simulink model "pacemaker_basic_model"  (R2020b)
settings: Solver=FixedStepAuto  StartTime=0.0  StopTime=10.0  FixedStep=1E-3  RelTol=1e-3  EnableMultiTasking=on
undefined symbols (not defined in the file): D0, D1, D10, D11, D12, D13, D2, D3, D4, D5, D6, D7, D8, D9, PTA0, PTA1, PTA2, PTB23, PTB9, PTC16, PTC17, PTC2, PTC3, PTC4, PTD0, PTD1, PTD2, PTD3
libraries: frdmk64flib x16
settings Model: ExtModeTrigDuration=5  Creator=Owner  LastModifiedBy=Anna
settings OptimizationCC: EnhancedBackFolding=on  PassReuseOutputArgsAs=Individual arguments  ZeroExternalMemoryAtStartup=off  ZeroInternalMemoryAtStartup=off  MaxStackSize=64  OptimizeBlockOrder=speed  DifferentSizesBufferReuse=on  OptimizationCustomize=off  EfficientTunableParamExpr=on
settings DebuggingCC: ParameterTunabilityLossMsg=error
settings HardwareCC: ProdBitPerPointer=32  ProdBitPerSizeT=32  ProdBitPerPtrDiffT=32  ProdLargestAtomicInteger=Long  ProdLargestAtomicFloat=Double  ProdWordSize=32  ProdHWDeviceType=ARM Compatible->ARM Cortex
settings SFSimCC: MATLABDynamicMemAlloc=off
settings RTWCC: Description=Embedded Coder  SystemTargetFile=ert.tlc  HardwareBoard=NXP FRDM-K64F  TLCOptions="-aInlineSetEventsForThisBaseRateFcn=TLC_FALSE -aSuppressMultiTaskScheduler=TLC_FALSE  -aRateBasedStepFcn=0"  TemplateMakefile=ert_default_tmf  Toolchain=GNU Tools for ARM Embedded Processors
settings CodeAppCC: ForceParamTrailComments=on  IgnoreCustomStorageClasses=off  OperatorAnnotations=on  SimulinkDataObjDesc=on  SFDataObjDesc=on  InsertBlockDesc=on
settings ERTTargetCC: ExtModeTransport=4  ExtModeMexFile=sendToCommService

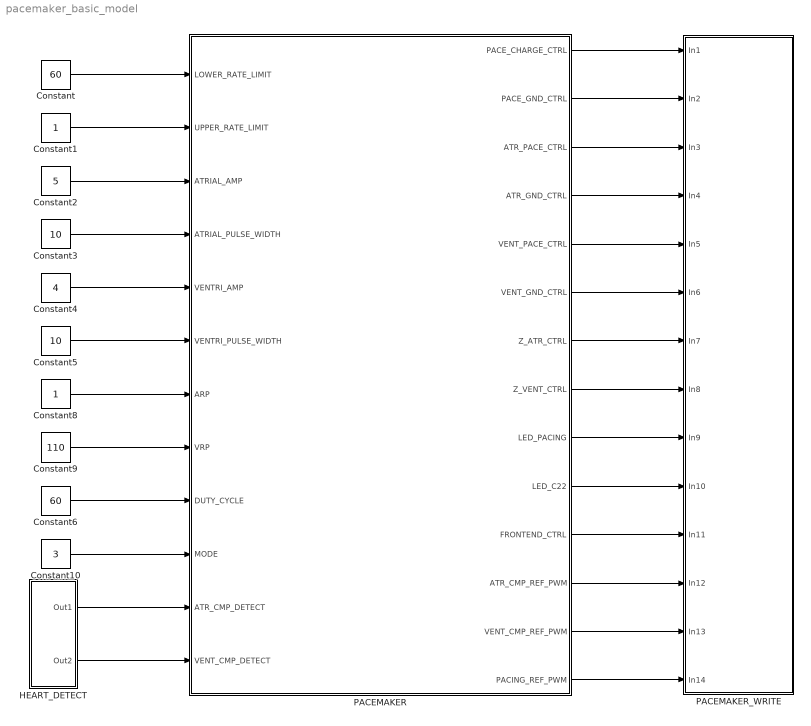
== system pacemaker_basic_model ==
  Constant : Constant  Value=60
  Constant1 : Constant
  Constant10 : Constant  Value=3
  Constant2 : Constant  Value=5
  Constant3 : Constant  Value=10
  Constant4 : Constant  Value=4
  Constant5 : Constant  Value=10
  Constant6 : Constant  Value=60
  Constant8 : Constant
  Constant9 : Constant  Value=110
  HEART_DETECT : Subsystem
  PACEMAKER : Stateflow chart  TreatAsAtomicUnit=on
  PACEMAKER_WRITE : Subsystem
  wires:
  Constant/1 -> PACEMAKER/1(LOWER_RATE_LIMIT)
  Constant1/1 -> PACEMAKER/2(UPPER_RATE_LIMIT)
  Constant2/1 -> PACEMAKER/3(ATRIAL_AMP)
  Constant3/1 -> PACEMAKER/4(ATRIAL_PULSE_WIDTH)
  Constant4/1 -> PACEMAKER/5(VENTRI_AMP)
  Constant5/1 -> PACEMAKER/6(VENTRI_PULSE_WIDTH)
  Constant8/1 -> PACEMAKER/7(ARP)
  Constant9/1 -> PACEMAKER/8(VRP)
  Constant10/1 -> PACEMAKER/10(MODE)
  Constant6/1 -> PACEMAKER/9(DUTY_CYCLE)
  PACEMAKER/1(PACE_CHARGE_CTRL) -> PACEMAKER_WRITE/1(In1)
  PACEMAKER/2(PACE_GND_CTRL) -> PACEMAKER_WRITE/2(In2)
  PACEMAKER/3(ATR_PACE_CTRL) -> PACEMAKER_WRITE/3(In3)
  PACEMAKER/4(ATR_GND_CTRL) -> PACEMAKER_WRITE/4(In4)
  PACEMAKER/5(VENT_PACE_CTRL) -> PACEMAKER_WRITE/5(In5)
  PACEMAKER/6(VENT_GND_CTRL) -> PACEMAKER_WRITE/6(In6)
  PACEMAKER/7(Z_ATR_CTRL) -> PACEMAKER_WRITE/7(In7)
  PACEMAKER/8(Z_VENT_CTRL) -> PACEMAKER_WRITE/8(In8)
  PACEMAKER/9(LED_PACING) -> PACEMAKER_WRITE/9(In9)
  PACEMAKER/10(LED_C22) -> PACEMAKER_WRITE/10(In10)
  PACEMAKER/11(FRONTEND_CTRL) -> PACEMAKER_WRITE/11(In11)
  PACEMAKER/12(ATR_CMP_REF_PWM) -> PACEMAKER_WRITE/12(In12)
  PACEMAKER/13(VENT_CMP_REF_PWM) -> PACEMAKER_WRITE/13(In13)
  PACEMAKER/14(PACING_REF_PWM) -> PACEMAKER_WRITE/14(In14)
  HEART_DETECT/1(Out1) -> PACEMAKER/11(ATR_CMP_DETECT)
  HEART_DETECT/2(Out2) -> PACEMAKER/12(VENT_CMP_DETECT)

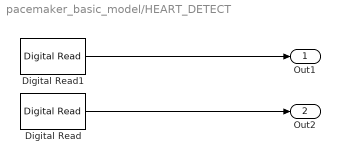
== system pacemaker_basic_model/HEART_DETECT ==
  Digital Read : frdmk64flib/Digital Read  Whichpin=PTC17 (D1)  SampleTime=-1
  Digital Read1 : frdmk64flib/Digital Read  Whichpin=PTC16 (D0)  SampleTime=-1
  Out1 : Outport
  Out2 : Outport  Port=2
  wires:
  Digital Read/1 -> Out2/1
  Digital Read1/1 -> Out1/1

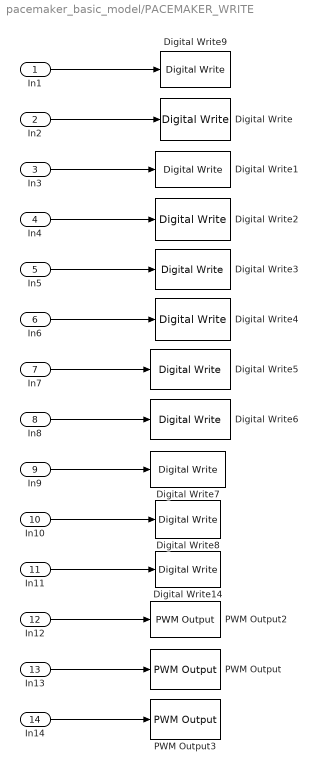
== system pacemaker_basic_model/PACEMAKER_WRITE ==
  In1 : Inport
  In2 : Inport  Port=2
  In3 : Inport  Port=3
  In4 : Inport  Port=4
  In5 : Inport  Port=5
  In6 : Inport  Port=6
  In7 : Inport  Port=7
  In8 : Inport  Port=8
  In9 : Inport  Port=9
  In10 : Inport  Port=10
  In11 : Inport  Port=11
  In12 : Inport  Port=12
  In13 : Inport  Port=13
  In14 : Inport  Port=14
  Digital Write : frdmk64flib/Digital Write  Whichpin=PTD0 (D10)
  Digital Write1 : frdmk64flib/Digital Write  Whichpin=PTA0 (D8)
  Digital Write14 : frdmk64flib/Digital Write  Whichpin=PTD1 (D13)
  Digital Write2 : frdmk64flib/Digital Write  Whichpin=PTD2 (D11)
  Digital Write3 : frdmk64flib/Digital Write  Whichpin=PTC4 (D9)
  Digital Write4 : frdmk64flib/Digital Write  Whichpin=PTD3 (D12)
  Digital Write5 : frdmk64flib/Digital Write  Whichpin=PTB23 (D4)
  Digital Write6 : frdmk64flib/Digital Write  Whichpin=PTC3 (D7)
  Digital Write7 : frdmk64flib/Digital Write  Whichpin=RED_LED
  Digital Write8 : frdmk64flib/Digital Write  Whichpin=BLUE_LED
  Digital Write9 : frdmk64flib/Digital Write  Whichpin=PTB9 (D2)
  PWM Output : frdmk64flib/PWM Output  Whichpin=PTA1 (D3)  InitialFrequency=2000  InitialDutyCycle=100
  PWM Output2 : frdmk64flib/PWM Output  Whichpin=PTC2 (D6)  InitialFrequency=2000  InitialDutyCycle=100
  PWM Output3 : frdmk64flib/PWM Output  Whichpin=PTA2 (D5)  InitialFrequency=2000  InitialDutyCycle=100
  wires:
  In10/1 -> Digital Write8/1
  In2/1 -> Digital Write/1
  In12/1 -> PWM Output2/1
  In7/1 -> Digital Write5/1
  In4/1 -> Digital Write2/1
  In8/1 -> Digital Write6/1
  In11/1 -> Digital Write14/1
  In1/1 -> Digital Write9/1
  In6/1 -> Digital Write4/1
  In9/1 -> Digital Write7/1
  In14/1 -> PWM Output3/1
  In3/1 -> Digital Write1/1
  In13/1 -> PWM Output/1
  In5/1 -> Digital Write3/1

== stateflow chart pacemaker_basic_model/PACEMAKER ==
  state MODE_VVI
    entry:
    FRONTEND_CTRL = true
    state VVI_CHARGING_SENSING
      entry:
      %Sensing Circuitry
      VENT_CMP_REF_PWM = DUTY_CYCLE
      ATR_CMP_REF_PWM = 0
      %Discharging C21
      PACE_GND_CTRL = true
      VENT_PACE_CTRL = false
      Z_ATR_CTRL = false
      Z_VENT_CTRL = false
      ATR_PACE_CTRL = false
      ATR_GND_CTRL = false
      VENT_GND_CTRL = true
      %Charging C22
      ATR_PACE_CTRL = false
      VENT_PACE_CTRL = false
      PACING_REF_PWM = 100*VENTRI_AMP/5
      PACE_CHARGE_CTRL = true
      LED_C22 = true
      exit:
      LED_C22 = false
    state PACE_READY
      entry:
      %Discharging C21
      PACE_GND_CTRL = true
      VENT_PACE_CTRL = false
      Z_ATR_CTRL = false
      Z_VENT_CTRL = false
      ATR_PACE_CTRL = false
      ATR_GND_CTRL = false
      VENT_GND_CTRL = true
      %Charging C22
      ATR_PACE_CTRL = false
      VENT_PACE_CTRL = false
      PACING_REF_PWM = 100*VENTRI_AMP/5
      PACE_CHARGE_CTRL = true
      LED_C22 = true
      exit:
      LED_C22 = false
    state PACING_VENTRICLE_VVI
      entry:
      PACE_CHARGE_CTRL = false
      PACE_GND_CTRL = true
      ATR_PACE_CTRL = false
      ATR_GND_CTRL = false
      Z_ATR_CTRL = false
      Z_VENT_CTRL = false
      VENT_GND_CTRL = false
      VENT_PACE_CTRL = true
      LED_PACING = true
      exit:
      LED_PACING = false
    VVI_CHARGING_SENSING -> PACING_VENTRICLE_VVI [order 1] : after(((60000/LOWER_RATE_LIMIT)-VENTRI_PULSE_WIDTH-VRP),msec) [VENT_CMP_DETECT== false]
    (default) -> VVI_CHARGING_SENSING
    MODE_VVI.PACE_READY -> VVI_CHARGING_SENSING : after(VRP, msec)
    PACING_VENTRICLE_VVI -> MODE_VVI.PACE_READY : after(VENTRI_PULSE_WIDTH, msec)
    VVI_CHARGING_SENSING -> MODE_VVI.PACE_READY [order 2] : [VENT_CMP_DETECT == true]
  state MODE_VOO
    entry:
    FRONTEND_CTRL = false
    state VOO_CHARGING
      entry:
      %Discharging C21
      PACE_GND_CTRL = true
      VENT_PACE_CTRL = false
      Z_ATR_CTRL = false
      Z_VENT_CTRL = false
      ATR_GND_CTRL = false
      ATR_PACE_CTRL = false
      VENT_GND_CTRL = true
      %Charging C22
      ATR_PACE_CTRL = false
      VENT_PACE_CTRL = false
      PACING_REF_PWM = 100*VENTRI_AMP/5
      PACE_CHARGE_CTRL = true
      LED_C22 = true
      exit:
      LED_C22 = false
    state PACING_VENTRICLE_VOO
      entry:
      PACE_CHARGE_CTRL = false
      PACE_GND_CTRL = true
      ATR_PACE_CTRL = false
      ATR_GND_CTRL = false
      Z_ATR_CTRL = false
      Z_VENT_CTRL = false
      VENT_GND_CTRL = false
      VENT_PACE_CTRL = true
      LED_PACING = true
      exit:
      LED_PACING = false
    PACING_VENTRICLE_VOO -> VOO_CHARGING : after(VENTRI_PULSE_WIDTH, msec)
    (default) -> VOO_CHARGING
    VOO_CHARGING -> PACING_VENTRICLE_VOO : after(((60000/LOWER_RATE_LIMIT)-VENTRI_PULSE_WIDTH), msec)
  state MODE_AAI
    entry:
    FRONTEND_CTRL = true
    state AAI_CHARGING_SENSING
      entry:
      %Sensing Circuitry
      VENT_CMP_REF_PWM = 0
      ATR_CMP_REF_PWM = DUTY_CYCLE
      %Discharging C21
      PACE_GND_CTRL = true
      VENT_PACE_CTRL = false
      Z_ATR_CTRL = false
      Z_VENT_CTRL = false
      ATR_PACE_CTRL = false
      ATR_GND_CTRL = true
      VENT_GND_CTRL = false
      %Charging C22
      ATR_PACE_CTRL = false
      VENT_PACE_CTRL = false
      PACING_REF_PWM = 100*ATRIAL_AMP/5
      PACE_CHARGE_CTRL = true
      LED_C22 = true
      exit:
      LED_C22 = false
    state PACE_READY
      entry:
      %Discharging C21
      PACE_GND_CTRL = true
      VENT_PACE_CTRL = false
      Z_ATR_CTRL = false
      Z_VENT_CTRL = false
      ATR_PACE_CTRL = false
      ATR_GND_CTRL = true
      VENT_GND_CTRL = false
      %Charging C22
      ATR_PACE_CTRL = false
      VENT_PACE_CTRL = false
      PACING_REF_PWM = 100*ATRIAL_AMP/5
      PACE_CHARGE_CTRL = true
      LED_C22 = true
      exit:
      LED_C22 = false
    state PACING_ATRIUM_AAI
      entry:
      PACE_CHARGE_CTRL = false
      PACE_GND_CTRL = true
      ATR_PACE_CTRL = true
      ATR_GND_CTRL = false
      Z_ATR_CTRL = false
      Z_VENT_CTRL = false
      VENT_GND_CTRL = false
      VENT_PACE_CTRL = false
      LED_PACING = true
      exit:
      LED_PACING = false
    AAI_CHARGING_SENSING -> PACING_ATRIUM_AAI [order 1] : after(((60000/LOWER_RATE_LIMIT)-ATRIAL_PULSE_WIDTH-ARP),msec) [ATR_CMP_DETECT== false]
    (default) -> AAI_CHARGING_SENSING
    MODE_AAI.PACE_READY -> AAI_CHARGING_SENSING : after(ARP, msec)
    PACING_ATRIUM_AAI -> MODE_AAI.PACE_READY : after(ATRIAL_PULSE_WIDTH, msec)
    AAI_CHARGING_SENSING -> MODE_AAI.PACE_READY [order 2] : [ATR_CMP_DETECT == true]
  state MODE_AOO
    entry:
    FRONTEND_CTRL = false
    state AOO_CHARGING
      entry:
      %Discharging C21
      PACE_GND_CTRL = true
      VENT_PACE_CTRL = false
      Z_ATR_CTRL = false
      Z_VENT_CTRL = false
      ATR_PACE_CTRL = false
      ATR_GND_CTRL = true
      VENT_GND_CTRL = false
      %Charging C22
      ATR_PACE_CTRL = false
      VENT_PACE_CTRL = false
      PACING_REF_PWM = 100*ATRIAL_AMP/5
      PACE_CHARGE_CTRL = true
      LED_C22 = true
      exit:
      LED_C22 = false
    state PACING_ATRIUM_AOO
      entry:
      PACE_CHARGE_CTRL = false
      PACE_GND_CTRL = true
      ATR_PACE_CTRL = true
      ATR_GND_CTRL = false
      Z_ATR_CTRL = false
      Z_VENT_CTRL = false
      VENT_GND_CTRL = false
      VENT_PACE_CTRL = false
      LED_PACING = true
      exit:
      LED_PACING = false
    AOO_CHARGING -> PACING_ATRIUM_AOO : after(((60000/LOWER_RATE_LIMIT)-ATRIAL_PULSE_WIDTH), msec)
    (default) -> AOO_CHARGING
    PACING_ATRIUM_AOO -> AOO_CHARGING : after(ATRIAL_PULSE_WIDTH, msec)
  (junction 79) -> MODE_VOO [order 1] : [MODE == 1]
  (junction 79) -> MODE_VVI [order 4]
  (default) -> (junction 79)
  (junction 79) -> MODE_AOO [order 2] : [MODE == 0]
  (junction 79) -> MODE_AAI [order 3] : [MODE == 2]
  data: PACE_CHARGE_CTRL output; PACE_GND_CTRL output; ATR_PACE_CTRL output; ATR_GND_CTRL output; VENT_PACE_CTRL output; VENT_GND_CTRL output; Z_ATR_CTRL output; Z_VENT_CTRL output; LED_PACING output; LED_C22 output; LOWER_RATE_LIMIT input; UPPER_RATE_LIMIT input; ATRIAL_AMP input; ATRIAL_PULSE_WIDTH input; VENTRI_AMP input; VENTRI_PULSE_WIDTH input; ARP input; VRP input; FRONTEND_CTRL output; ATR_CMP_REF_PWM output; VENT_CMP_REF_PWM output; PACING_REF_PWM output; DUTY_CYCLE input; MODE input; ATR_CMP_DETECT input; VENT_CMP_DETECT input
